simulink model "model_b"  (R2024b)
settings: Solver=ode4  StartTime=0.0  StopTime=simTime  FixedStep=sample_time  RelTol=1e-3
values from neighbouring files (symbols this model uses):
  a_m = 1    [init.m]
  b = 1    [init.m]    (also in init_a.m = 10*rand(1); init_b.m = 10*rand(1); init_ca.m; init_cb.m)
  gamma = 6    [init.m]    (also in init_a.m = 1; init_b.m = 1; init_ca.m = 1; init_cb.m = 1)
  sineAmp = 1    [init_a.m]    (also in init_b.m; init_ca.m; init_cb.m; init_d.m)
settings Model: Creator=kemal  LastModifiedBy=kemal

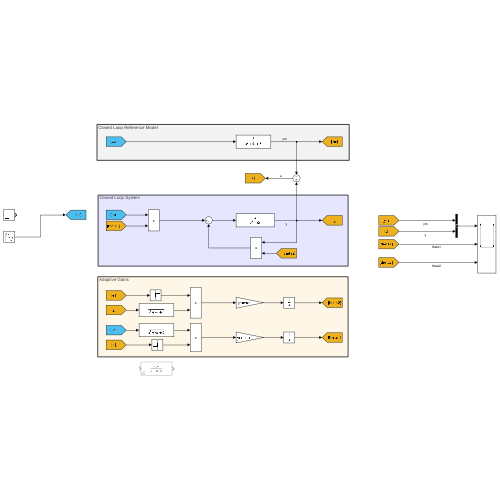
[thumbnail: Simulink's stored preview of the top-level diagram]
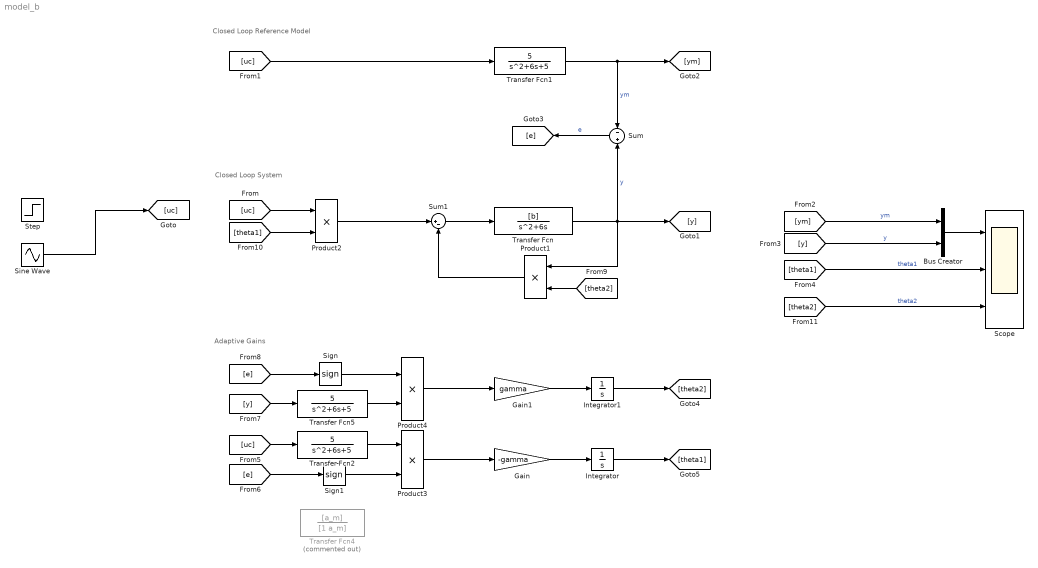
== system model_b ==
  note: Closed Loop Reference Model
  note: Adaptive Gains
  note: Closed Loop System
  Bus Creator : BusCreator  Inputs=2
  Gain : Gain  Gain=-gamma
  Gain1 : Gain  Gain=gamma
  Integrator : Integrator
  Integrator1 : Integrator
  Product{1..4} (4 alike) : Product
  Scope : Scope  NumInputPorts=3
  Sign : Signum
  Sign1 : Signum
  Sine Wave : Sin  Amplitude=sineAmp  Frequency=2*pi/5  SampleTime=0
  Step : Step  SampleTime=0
  Sum : Sum  Inputs=-+
  Sum1 : Sum  Inputs=|+-
  Transfer Fcn : TransferFcn  Numerator=[b]  Denominator=[1 6 0]
  Transfer Fcn1 : TransferFcn  Numerator=[5]  Denominator=[1 6 5]
  Transfer Fcn2 : TransferFcn  Numerator=[5]  Denominator=[1 6 5]
  Transfer Fcn4 : TransferFcn  Commented=on  Numerator=[a_m]  Denominator=[1 a_m]
  Transfer Fcn5 : TransferFcn  Numerator=[5]  Denominator=[1 6 5]
  wires:
  [uc] -> Transfer Fcn1/1
  Transfer Fcn1/1 -> [ym], Sum/1  "ym"
  Transfer Fcn/1 -> Product1/1, Sum/2, [y]  "y"
  Sine Wave/1 -> [uc]
  [ym] -> Bus Creator/1  "ym"
  [y] -> Bus Creator/2  "y"
  Bus Creator/1 -> Scope/1
  [theta1] -> Scope/2  "theta1"
  Sum1/1 -> Transfer Fcn/1
  Product1/1 -> Sum1/2
  [uc] -> Product2/1
  Product2/1 -> Sum1/1
  Sum/1 -> [e]  "e"
  Integrator/1 -> [theta1]
  Gain/1 -> Integrator/1
  [uc] -> Transfer Fcn2/1
  Transfer Fcn2/1 -> Product3/1
  [e] -> Sign1/1
  Product3/1 -> Gain/1
  [y] -> Transfer Fcn5/1
  Gain1/1 -> Integrator1/1
  Transfer Fcn5/1 -> Product4/2
  [e] -> Sign/1
  Product4/1 -> Gain1/1
  Integrator1/1 -> [theta2]
  [theta2] -> Product1/2
  [theta1] -> Product2/2
  [theta2] -> Scope/3  "theta2"
  Sign/1 -> Product4/1
  Sign1/1 -> Product3/2
